simulink model "simulink_group17"  (R2023b)
settings: Solver=FixedStepAuto  StartTime=0.0  StopTime=10.0  FixedStep=1e-3  RelTol=1e-3  EnableMultiTasking=on
undefined symbols (not defined in the file): D0, D1, D10, D11, D12, D13, D2, D3, D4, D5, D6, D7, D8, D9, PTA0, PTA1, PTA2, PTB23, PTB9, PTC16, PTC17, PTC2, PTC3, PTC4, PTD0, PTD1, PTD2, PTD3
libraries: frdmk64flib x15
settings Model: ExtModeTrigDuration=5  Creator=ow  LastModifiedBy=reemb
settings SolverCC: AlgebraicLoopSolver=TrustRegion
settings OptimizationCC: EnhancedBackFolding=on  PassReuseOutputArgsAs=Individual arguments  ZeroExternalMemoryAtStartup=off  ZeroInternalMemoryAtStartup=off  MaxStackSize=64  OptimizeBlockOrder=speed  DifferentSizesBufferReuse=on  OptimizationCustomize=off  EfficientTunableParamExpr=on
settings DebuggingCC: ParameterTunabilityLossMsg=error  UnconnectedInputMsg=warning  UnconnectedOutputMsg=warning  UnconnectedLineMsg=warning
settings HardwareCC: ProdBitPerPointer=32  ProdBitPerSizeT=32  ProdBitPerPtrDiffT=32  ProdLargestAtomicInteger=Long  ProdLargestAtomicFloat=Double  ProdWordSize=32  ProdHWDeviceType=ARM Compatible->ARM Cortex
settings ModelReferenceCC: EnableRefExpFcnMdlSchedulingChecks=on
settings SFSimCC: MATLABDynamicMemAlloc=off
settings RTWCC: Description=Embedded Coder  SystemTargetFile=ert.tlc  HardwareBoard=NXP FRDM-K64F  TLCOptions="-aInlineSetEventsForThisBaseRateFcn=TLC_FALSE -aSuppressMultiTaskScheduler=TLC_FALSE  -aRateBasedStepFcn=0"  TemplateMakefile=ert_default_tmf  Toolchain=GNU Tools for ARM Embedded Processors
settings CodeAppCC: ForceParamTrailComments=on  IgnoreCustomStorageClasses=off  OperatorAnnotations=on  SimulinkDataObjDesc=on  SFDataObjDesc=on  InsertBlockDesc=on

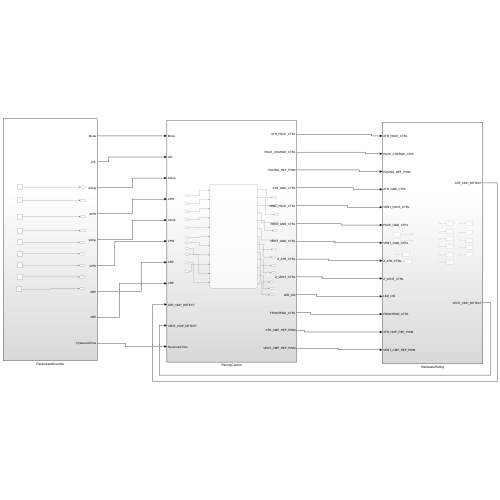
[thumbnail: Simulink's stored preview of the top-level diagram]
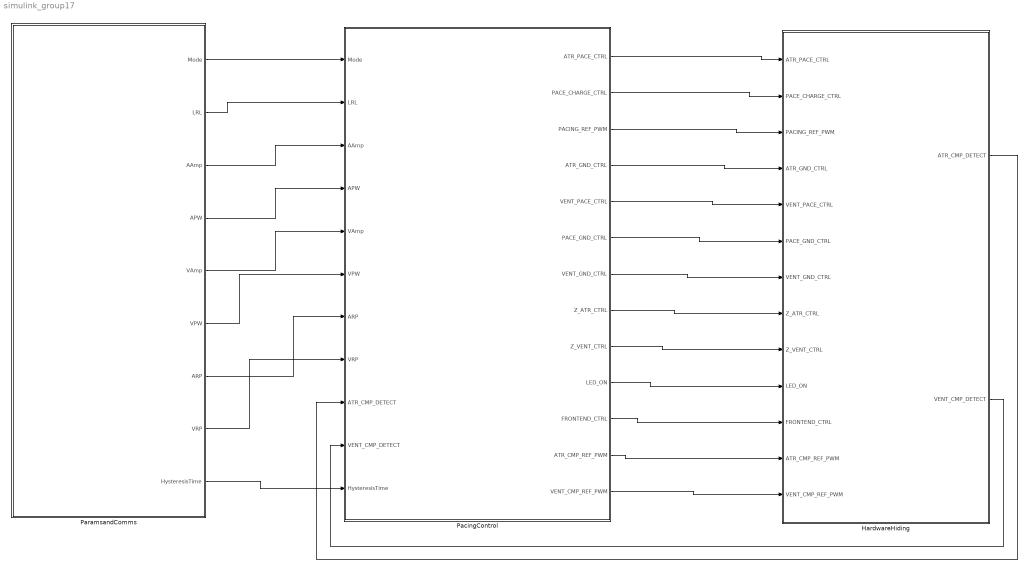
== system simulink_group17 ==
  HardwareHiding : Subsystem
  PacingControl : Subsystem
  ParamsandComms : Subsystem
  wires:
  ParamsandComms/1(Mode) -> PacingControl/1(Mode)
  ParamsandComms/2(LRL) -> PacingControl/2(LRL)
  ParamsandComms/3(AAmp) -> PacingControl/3(AAmp)
  ParamsandComms/4(APW) -> PacingControl/4(APW)
  ParamsandComms/6(VPW) -> PacingControl/6(VPW)
  ParamsandComms/5(VAmp) -> PacingControl/5(VAmp)
  ParamsandComms/7(ARP) -> PacingControl/7(ARP)
  ParamsandComms/8(VRP) -> PacingControl/8(VRP)
  PacingControl/1(ATR_PACE_CTRL) -> HardwareHiding/1(ATR_PACE_CTRL)
  PacingControl/2(PACE_CHARGE_CTRL) -> HardwareHiding/2(PACE_CHARGE_CTRL)
  PacingControl/3(PACING_REF_PWM) -> HardwareHiding/3(PACING_REF_PWM)
  PacingControl/5(VENT_PACE_CTRL) -> HardwareHiding/5(VENT_PACE_CTRL)
  PacingControl/4(ATR_GND_CTRL) -> HardwareHiding/4(ATR_GND_CTRL)
  PacingControl/6(PACE_GND_CTRL) -> HardwareHiding/6(PACE_GND_CTRL)
  PacingControl/7(VENT_GND_CTRL) -> HardwareHiding/7(VENT_GND_CTRL)
  PacingControl/8(Z_ATR_CTRL) -> HardwareHiding/8(Z_ATR_CTRL)
  PacingControl/9(Z_VENT_CTRL) -> HardwareHiding/9(Z_VENT_CTRL)
  PacingControl/10(LED_ON) -> HardwareHiding/10(LED_ON)
  PacingControl/11(FRONTEND_CTRL) -> HardwareHiding/11(FRONTEND_CTRL)
  ParamsandComms/9(HysteresisTime) -> PacingControl/11(HysteresisTime)
  HardwareHiding/1(ATR_CMP_DETECT) -> PacingControl/9(ATR_CMP_DETECT)
  HardwareHiding/2(VENT_CMP_DETECT) -> PacingControl/10(VENT_CMP_DETECT)
  PacingControl/12(ATR_CMP_REF_PWM) -> HardwareHiding/12(ATR_CMP_REF_PWM)
  PacingControl/13(VENT_CMP_REF_PWM) -> HardwareHiding/13(VENT_CMP_REF_PWM)

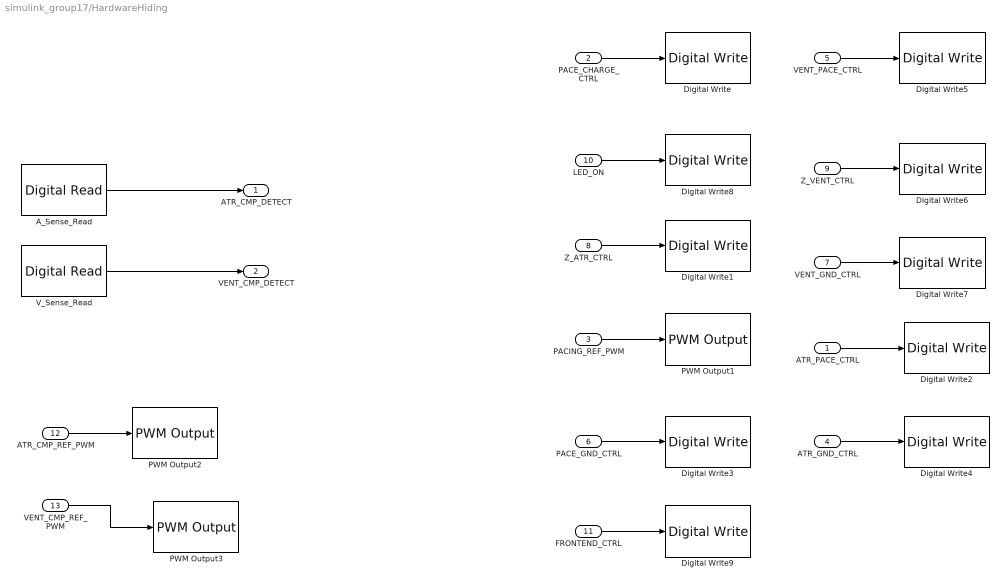
== system simulink_group17/HardwareHiding ==
  ATR_PACE_CTRL : Inport
  PACE_CHARGE_CTRL : Inport  Port=2
  PACING_REF_PWM : Inport  Port=3
  ATR_GND_CTRL : Inport  Port=4
  VENT_PACE_CTRL : Inport  Port=5
  PACE_GND_CTRL : Inport  Port=6
  VENT_GND_CTRL : Inport  Port=7
  Z_ATR_CTRL : Inport  Port=8
  Z_VENT_CTRL : Inport  Port=9
  LED_ON : Inport  Port=10
  FRONTEND_CTRL : Inport  Port=11
  ATR_CMP_REF_PWM : Inport  Port=12
  VENT_CMP_REF_PWM : Inport  Port=13
  A_Sense_Read : frdmk64flib/Digital Read  Whichpin=PTC16 (D0)  SampleTime=-1
  Digital Write : frdmk64flib/Digital Write  Whichpin=PTB9 (D2)
  Digital Write1 : frdmk64flib/Digital Write  Whichpin=PTB23 (D4)
  Digital Write2 : frdmk64flib/Digital Write  Whichpin=PTA0 (D8)
  Digital Write3 : frdmk64flib/Digital Write  Whichpin=PTD0 (D10)
  Digital Write4 : frdmk64flib/Digital Write  Whichpin=PTD2 (D11)
  Digital Write5 : frdmk64flib/Digital Write  Whichpin=PTC4 (D9)
  Digital Write6 : frdmk64flib/Digital Write  Whichpin=PTC3 (D7)
  Digital Write7 : frdmk64flib/Digital Write  Whichpin=PTD3 (D12)
  Digital Write8 : frdmk64flib/Digital Write  Whichpin=RED_LED
  Digital Write9 : frdmk64flib/Digital Write  Whichpin=PTD1 (D13)
  PWM Output1 : frdmk64flib/PWM Output  Whichpin=PTA2 (D5)  InitialFrequency=2000  InitialDutyCycle=50
  PWM Output2 : frdmk64flib/PWM Output  Whichpin=PTC2 (D6)  InitialFrequency=2000  InitialDutyCycle=100
  PWM Output3 : frdmk64flib/PWM Output  Whichpin=PTA1 (D3)  InitialFrequency=2000  InitialDutyCycle=100
  V_Sense_Read : frdmk64flib/Digital Read  Whichpin=PTC17 (D1)  SampleTime=-1
  ATR_CMP_DETECT : Outport
  VENT_CMP_DETECT : Outport  Port=2
  wires:
  A_Sense_Read/1 -> ATR_CMP_DETECT/1
  V_Sense_Read/1 -> VENT_CMP_DETECT/1
  Z_VENT_CTRL/1 -> Digital Write6/1
  LED_ON/1 -> Digital Write8/1
  ATR_PACE_CTRL/1 -> Digital Write2/1
  Z_ATR_CTRL/1 -> Digital Write1/1
  VENT_GND_CTRL/1 -> Digital Write7/1
  PACE_CHARGE_CTRL/1 -> Digital Write/1
  PACE_GND_CTRL/1 -> Digital Write3/1
  PACING_REF_PWM/1 -> PWM Output1/1
  VENT_PACE_CTRL/1 -> Digital Write5/1
  ATR_GND_CTRL/1 -> Digital Write4/1
  FRONTEND_CTRL/1 -> Digital Write9/1
  ATR_CMP_REF_PWM/1 -> PWM Output2/1
  VENT_CMP_REF_PWM/1 -> PWM Output3/1

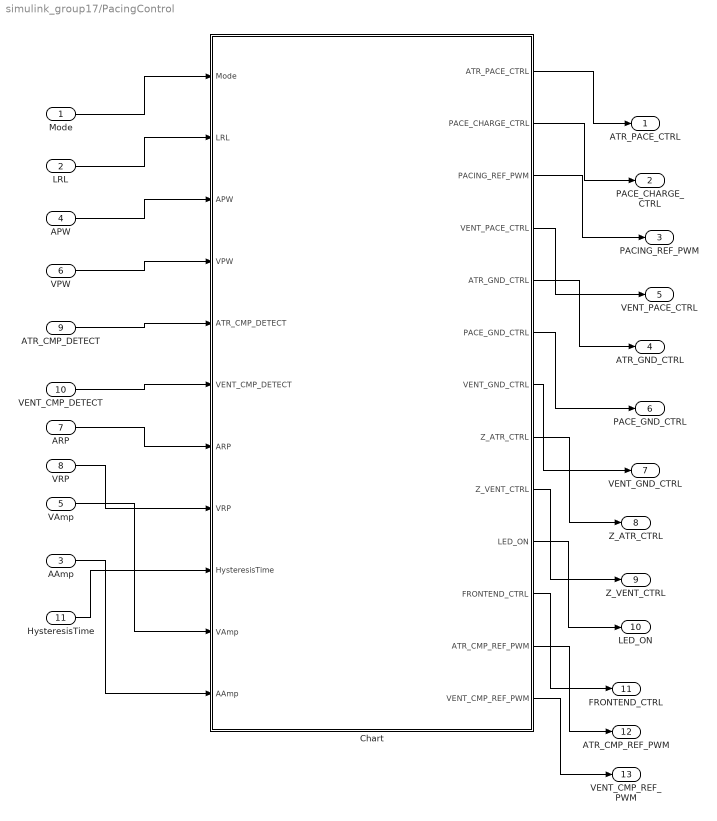
== system simulink_group17/PacingControl ==
  Mode : Inport
  LRL : Inport  Port=2
  AAmp : Inport  Port=3
  APW : Inport  Port=4
  VAmp : Inport  Port=5
  VPW : Inport  Port=6
  ARP : Inport  Port=7
  VRP : Inport  Port=8
  ATR_CMP_DETECT : Inport  Port=9
  VENT_CMP_DETECT : Inport  Port=10
  HysteresisTime : Inport  Port=11
  Chart : Stateflow chart  TreatAsAtomicUnit=on
      settings: PortSchema="{\"entries\":[{\"content\":{\"sides\":[{\"content\":{\"connectorIds\":[\"In1\",\"In2\",\"In5\",\"In3\",\"In4\",\"In6\",\"In7\",\"In10\",\"In11\",\"In8\",\"In9\"]},\"type\":\"ConnectorPlacement.EquallySpacedRectSide\",\"uuid\":\"2cabd690-10ca-439e-b217-62815d125176\"},{\"content\":{\"connectorIds\":[\"Out1\",\"Out2\",\"Out3\",\"Out4\",\"Out5\",\"Out6\",\"Out7\",\"Out8\",\"Out9\",\"Out10\",\"Out11\",\"Out12\",\"Out13\"],\"side\":\"RIGHT\"},\"type\":\"ConnectorPlacement.EquallySpacedRectSide\",\"uuid\":\"e8964e9d-7b02-47f5-a48a-30c87640778e\"},{\"content\":{\"side\":\"TOP\"},\"type\":\"ConnectorPlacement.EquallySpacedRectSide\",\"uuid\":\"37da63f5-52a1-4b9c-b728-2e179414b5fa\"}]},\"type\":\"ConnectorPlacement.EquallySpacedConnector\",\"uuid\":\"fe4480b5-e88f-4b9f-8d05-cd2d47a8a31d\"}],\"packageUris\":[\"http://schema.mathworks.com/mf0/Connector/R2020b\"],\"version\":\"1.0\"}"
  ATR_PACE_CTRL : Outport
  PACE_CHARGE_CTRL : Outport  Port=2
  PACING_REF_PWM : Outport  Port=3
  ATR_GND_CTRL : Outport  Port=4
  VENT_PACE_CTRL : Outport  Port=5
  PACE_GND_CTRL : Outport  Port=6
  VENT_GND_CTRL : Outport  Port=7
  Z_ATR_CTRL : Outport  Port=8
  Z_VENT_CTRL : Outport  Port=9
  LED_ON : Outport  Port=10
  FRONTEND_CTRL : Outport  Port=11
  ATR_CMP_REF_PWM : Outport  Port=12
  VENT_CMP_REF_PWM : Outport  Port=13
  wires:
  LRL/1 -> Chart/2(LRL)
  Mode/1 -> Chart/1(Mode)
  VPW/1 -> Chart/3(VPW)
  ATR_CMP_DETECT/1 -> Chart/4(ATR_CMP_DETECT)
  APW/1 -> Chart/5(APW)
  ARP/1 -> Chart/7(ARP)
  VRP/1 -> Chart/10(VRP)
  AAmp/1 -> Chart/9(AAmp)
  VAmp/1 -> Chart/8(VAmp)
  Chart/1(ATR_PACE_CTRL) -> ATR_PACE_CTRL/1
  Chart/2(PACE_CHARGE_CTRL) -> PACE_CHARGE_CTRL/1
  Chart/3(PACING_REF_PWM) -> PACING_REF_PWM/1
  Chart/5(ATR_GND_CTRL) -> ATR_GND_CTRL/1
  Chart/6(PACE_GND_CTRL) -> PACE_GND_CTRL/1
  Chart/7(VENT_GND_CTRL) -> VENT_GND_CTRL/1
  Chart/8(Z_ATR_CTRL) -> Z_ATR_CTRL/1
  Chart/9(Z_VENT_CTRL) -> Z_VENT_CTRL/1
  Chart/11(FRONTEND_CTRL) -> FRONTEND_CTRL/1
  HysteresisTime/1 -> Chart/11(HysteresisTime)
  Chart/4(VENT_PACE_CTRL) -> VENT_PACE_CTRL/1
  Chart/10(LED_ON) -> LED_ON/1
  VENT_CMP_DETECT/1 -> Chart/6(VENT_CMP_DETECT)
  Chart/12(ATR_CMP_REF_PWM) -> ATR_CMP_REF_PWM/1
  Chart/13(VENT_CMP_REF_PWM) -> VENT_CMP_REF_PWM/1

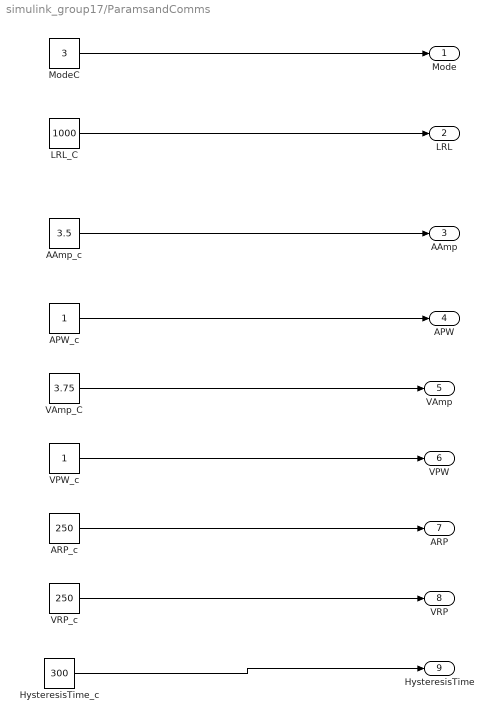
== system simulink_group17/ParamsandComms ==
  AAmp_c : Constant  Value=3.5
  APW_c : Constant
  ARP_c : Constant  Value=250
  HysteresisTime_c : Constant  Value=300
  LRL_C : Constant  Value=1000  SampleTime=-1
  ModeC : Constant  Value=3
  VAmp_C : Constant  Value=3.75
  VPW_c : Constant
  VRP_c : Constant  Value=250
  Mode : Outport
  LRL : Outport  Port=2
  AAmp : Outport  Port=3
  APW : Outport  Port=4
  VAmp : Outport  Port=5
  VPW : Outport  Port=6
  ARP : Outport  Port=7
  VRP : Outport  Port=8
  HysteresisTime : Outport  Port=9
  wires:
  ModeC/1 -> Mode/1
  LRL_C/1 -> LRL/1
  AAmp_c/1 -> AAmp/1
  APW_c/1 -> APW/1
  VRP_c/1 -> VRP/1
  ARP_c/1 -> ARP/1
  VPW_c/1 -> VPW/1
  VAmp_C/1 -> VAmp/1
  HysteresisTime_c/1 -> HysteresisTime/1

== stateflow chart simulink_group17/PacingControl/Chart ==
  state AAI
    state ChargingDischarging
      entry:
      %Enable Sensing
      FRONTEND_CTRL = 1;
      ATR_CMP_REF_PWM = 90;
      %Charging
      PACE_CHARGE_CTRL = 1;
      ATR_PACE_CTRL = 0;
      VENT_PACE_CTRL = 0;
      PACING_REF_PWM = (AAmp/5) * 100;
      %Discharging
      PACE_GND_CTRL = 1;
      ATR_PACE_CTRL = 0;
      ATR_GND_CTRL = 1;
      VENT_PACE_CTRL = 0;
      VENT_GND_CTRL = 0;
      Z_ATR_CTRL = 0;
      Z_VENT_CTRL = 0;
      LED_ON = 0;
    state Pacing
      entry:
      %Disable Sensing
      FRONTEND_CTRL = 0;
      %Pace Ventricle
      PACE_CHARGE_CTRL = 0;
      PACE_GND_CTRL = 1;
      ATR_PACE_CTRL = 1;
      ATR_GND_CTRL = 0;
      VENT_PACE_CTRL = 0;
      VENT_GND_CTRL = 0;
      Z_ATR_CTRL = 0;
      Z_VENT_CTRL = 0;
      LED_ON = 1;
    state Hysteresis
      entry:
      %Enable Sensing
      FRONTEND_CTRL = 1;
      %Charging
      PACE_CHARGE_CTRL = 1;
      ATR_PACE_CTRL = 0;
      VENT_PACE_CTRL = 0;
      %Discharging
      PACE_GND_CTRL = 1;
      ATR_PACE_CTRL = 0;
      ATR_GND_CTRL = 1;
      VENT_PACE_CTRL = 0;
      VENT_GND_CTRL = 0;
      Z_ATR_CTRL = 0;
      Z_VENT_CTRL = 0;
      LED_ON = 0;
    (default) -> AAI.ChargingDischarging
    AAI.ChargingDischarging -> AAI.Pacing [order 1] : [after(LRL- ARP, msec) ]
    AAI.Pacing -> AAI.ChargingDischarging : [after(APW,msec)]
    AAI.Hysteresis -> AAI.Pacing [order 2] : [after(LRL + HysteresisTime, msec)]
    AAI.Hysteresis -> AAI.ChargingDischarging [order 3] : [after(ARP, msec)]
    AAI.ChargingDischarging -> AAI.Hysteresis [order 2] : [ ATR_CMP_DETECT==1]
    AAI.Hysteresis -> AAI.Hysteresis [order 1] : [after(ARP, msec) && ATR_CMP_DETECT==1]
  state VVI
    state ChargingDischarging
      entry:
      %Enable Sensing
      FRONTEND_CTRL = 1;
      VENT_CMP_REF_PWM = 90;
      %Charging
      PACE_CHARGE_CTRL = 1;
      ATR_PACE_CTRL = 0;
      VENT_PACE_CTRL = 0;
      PACING_REF_PWM = (VAmp/5) * 100;
      %Discharging
      PACE_GND_CTRL = 1;
      ATR_PACE_CTRL = 0;
      ATR_GND_CTRL = 0;
      VENT_PACE_CTRL = 0;
      VENT_GND_CTRL = 1;
      Z_ATR_CTRL = 0;
      Z_VENT_CTRL = 0;
      LED_ON = 0;
    state VPacing
      entry:
      %Disable Sensing
      FRONTEND_CTRL = 0;
      %Pace Ventricle
      PACE_CHARGE_CTRL = 0;
      PACE_GND_CTRL = 1;
      ATR_PACE_CTRL = 0;
      ATR_GND_CTRL = 0;
      VENT_PACE_CTRL = 1;
      VENT_GND_CTRL = 0;
      Z_ATR_CTRL = 0;
      Z_VENT_CTRL = 0;
      LED_ON = 1;
    state Hysteresis
      entry:
      %Enable Sensing
      FRONTEND_CTRL = 1;
      %Charging
      PACE_CHARGE_CTRL = 1;
      ATR_PACE_CTRL = 0;
      VENT_PACE_CTRL = 0;
      %Discharging
      PACE_GND_CTRL = 1;
      ATR_PACE_CTRL = 0;
      ATR_GND_CTRL = 0;
      VENT_PACE_CTRL = 0;
      VENT_GND_CTRL = 1;
      Z_ATR_CTRL = 0;
      Z_VENT_CTRL = 0;
      LED_ON = 0;
    (default) -> VVI.ChargingDischarging
    VVI.ChargingDischarging -> VVI.VPacing [order 1] : [after(LRL-VRP, msec) ]
    VVI.VPacing -> VVI.ChargingDischarging : [after(VPW,msec)]
    VVI.Hysteresis -> VVI.VPacing [order 2] : [after(LRL + HysteresisTime, msec)]
    VVI.Hysteresis -> VVI.ChargingDischarging [order 3] : [after(VRP, msec)]
    VVI.ChargingDischarging -> VVI.Hysteresis [order 2] : [ VENT_CMP_DETECT==1]
    VVI.Hysteresis -> VVI.Hysteresis [order 1] : [after(VRP, msec) && VENT_CMP_DETECT==1]
  state AOO
    state APacing
      entry:
      %Pace Atrial
      PACE_CHARGE_CTRL = 0;
      PACE_GND_CTRL = 1;
      ATR_PACE_CTRL = 1;
      ATR_GND_CTRL = 0;
      VENT_PACE_CTRL = 0;
      VENT_GND_CTRL = 0;
      Z_ATR_CTRL = 0;
      Z_VENT_CTRL = 0;
      LED_ON = 1;
    state ChargingDischarging
      entry:
      %No Sensing
      FRONTEND_CTRL = 0;
      %Charging
      PACE_CHARGE_CTRL = 1;
      ATR_PACE_CTRL = 0;
      VENT_PACE_CTRL = 0;
      PACING_REF_PWM = (AAmp/5) * 100;
      %Discharging
      PACE_GND_CTRL = 1;
      ATR_PACE_CTRL = 0;
      ATR_GND_CTRL = 1;
      VENT_PACE_CTRL = 0;
      VENT_GND_CTRL = 0;
      Z_ATR_CTRL = 0;
      Z_VENT_CTRL = 0;
      LED_ON = 0;
    (default) -> state26
    AOO.APacing -> state26 : [after(APW,msec)]
    state26 -> AOO.APacing : [after(LRL-APW,msec)]
  state VOO
    state Chargin_Discharging
      entry:
      %No Sensing
      FRONTEND_CTRL = 0;
      %Charging
      PACE_CHARGE_CTRL = 1;
      ATR_PACE_CTRL = 0;
      VENT_PACE_CTRL = 0;
      PACING_REF_PWM = (VAmp/5) * 100;
      %Discharging
      PACE_GND_CTRL = 1;
      ATR_PACE_CTRL = 0;
      ATR_GND_CTRL = 0;
      VENT_PACE_CTRL = 0;
      VENT_GND_CTRL = 1;
      Z_ATR_CTRL = 0;
      Z_VENT_CTRL = 0;
      LED_ON = 0;
    state Pacing
      entry:
      %Pace Ventricle
      PACE_CHARGE_CTRL = 0;
      PACE_GND_CTRL = 1;
      ATR_PACE_CTRL = 0;
      ATR_GND_CTRL = 0;
      VENT_PACE_CTRL = 1;
      VENT_GND_CTRL = 0;
      Z_ATR_CTRL = 0;
      Z_VENT_CTRL = 0;
      LED_ON = 1;
    (default) -> VOO.Chargin_Discharging
    VOO.Chargin_Discharging -> VOO.Pacing : [after(LRL-VPW,msec)]
    VOO.Pacing -> VOO.Chargin_Discharging : [after(VPW,msec)]
  state InitialState
  state VVIR
    state ChargingDischarging
      entry:
      %Enable Sensing
      FRONTEND_CTRL = 1;
      VENT_CMP_REF_PWM = 90;
      %Charging
      PACE_CHARGE_CTRL = 1;
      ATR_PACE_CTRL = 0;
      VENT_PACE_CTRL = 0;
      PACING_REF_PWM = (VAmp/5) * 100;
      %Discharging
      PACE_GND_CTRL = 1;
      ATR_PACE_CTRL = 0;
      ATR_GND_CTRL = 0;
      VENT_PACE_CTRL = 0;
      VENT_GND_CTRL = 1;
      Z_ATR_CTRL = 0;
      Z_VENT_CTRL = 0;
      LED_ON = 0;
    state VPacing
      entry:
      %Disable Sensing
      FRONTEND_CTRL = 0;
      %Pace Ventricle
      PACE_CHARGE_CTRL = 0;
      PACE_GND_CTRL = 1;
      ATR_PACE_CTRL = 0;
      ATR_GND_CTRL = 0;
      VENT_PACE_CTRL = 1;
      VENT_GND_CTRL = 0;
      Z_ATR_CTRL = 0;
      Z_VENT_CTRL = 0;
      LED_ON = 1;
    state Hysteresis
      entry:
      %Enable Sensing
      FRONTEND_CTRL = 1;
      %Charging
      PACE_CHARGE_CTRL = 1;
      ATR_PACE_CTRL = 0;
      VENT_PACE_CTRL = 0;
      %Discharging
      PACE_GND_CTRL = 1;
      ATR_PACE_CTRL = 0;
      ATR_GND_CTRL = 0;
      VENT_PACE_CTRL = 0;
      VENT_GND_CTRL = 1;
      Z_ATR_CTRL = 0;
      Z_VENT_CTRL = 0;
      LED_ON = 0;
    (default) -> VVIR.ChargingDischarging
    VVIR.ChargingDischarging -> VVIR.VPacing [order 1] : [after(LRL-VRP, msec) ]
    VVIR.VPacing -> VVIR.ChargingDischarging : [after(VPW,msec)]
    VVIR.Hysteresis -> VVIR.VPacing [order 2] : [after(LRL + HysteresisTime, msec)]
    VVIR.Hysteresis -> VVIR.ChargingDischarging [order 3] : [after(VRP, msec)]
    VVIR.ChargingDischarging -> VVIR.Hysteresis [order 2] : [ VENT_CMP_DETECT==1]
    VVIR.Hysteresis -> VVIR.Hysteresis [order 1] : [after(VRP, msec) && VENT_CMP_DETECT==1]
  state AOOR
    state APacing
      entry:
      %Pace Atrial
      PACE_CHARGE_CTRL = 0;
      PACE_GND_CTRL = 1;
      ATR_PACE_CTRL = 1;
      ATR_GND_CTRL = 0;
      VENT_PACE_CTRL = 0;
      VENT_GND_CTRL = 0;
      Z_ATR_CTRL = 0;
      Z_VENT_CTRL = 0;
      LED_ON = 1;
    state ChargingDischarging
      entry:
      %No Sensing
      FRONTEND_CTRL = 0;
      %Charging
      PACE_CHARGE_CTRL = 1;
      ATR_PACE_CTRL = 0;
      VENT_PACE_CTRL = 0;
      PACING_REF_PWM = (AAmp/5) * 100;
      %Discharging
      PACE_GND_CTRL = 1;
      ATR_PACE_CTRL = 0;
      ATR_GND_CTRL = 1;
      VENT_PACE_CTRL = 0;
      VENT_GND_CTRL = 0;
      Z_ATR_CTRL = 0;
      Z_VENT_CTRL = 0;
      LED_ON = 0;
    note: % Switch out LRL in the transition with wtvr accelerometer variable you have (for all 4 new modes)
    (default) -> AOOR.ChargingDischarging
    AOOR.APacing -> AOOR.ChargingDischarging : [after(APW,msec)]
    AOOR.ChargingDischarging -> AOOR.APacing : [after(LRL-APW,msec)]
  state AAIR
    state ChargingDischarging
      entry:
      %Enable Sensing
      FRONTEND_CTRL = 1;
      ATR_CMP_REF_PWM = 90;
      %Charging
      PACE_CHARGE_CTRL = 1;
      ATR_PACE_CTRL = 0;
      VENT_PACE_CTRL = 0;
      PACING_REF_PWM = (AAmp/5) * 100;
      %Discharging
      PACE_GND_CTRL = 1;
      ATR_PACE_CTRL = 0;
      ATR_GND_CTRL = 1;
      VENT_PACE_CTRL = 0;
      VENT_GND_CTRL = 0;
      Z_ATR_CTRL = 0;
      Z_VENT_CTRL = 0;
      LED_ON = 0;
    state Pacing
      entry:
      %Disable Sensing
      FRONTEND_CTRL = 0;
      %Pace Ventricle
      PACE_CHARGE_CTRL = 0;
      PACE_GND_CTRL = 1;
      ATR_PACE_CTRL = 1;
      ATR_GND_CTRL = 0;
      VENT_PACE_CTRL = 0;
      VENT_GND_CTRL = 0;
      Z_ATR_CTRL = 0;
      Z_VENT_CTRL = 0;
      LED_ON = 1;
    state Hysteresis
      entry:
      %Enable Sensing
      FRONTEND_CTRL = 1;
      %Charging
      PACE_CHARGE_CTRL = 1;
      ATR_PACE_CTRL = 0;
      VENT_PACE_CTRL = 0;
      %Discharging
      PACE_GND_CTRL = 1;
      ATR_PACE_CTRL = 0;
      ATR_GND_CTRL = 1;
      VENT_PACE_CTRL = 0;
      VENT_GND_CTRL = 0;
      Z_ATR_CTRL = 0;
      Z_VENT_CTRL = 0;
      LED_ON = 0;
    (default) -> AAIR.ChargingDischarging
    AAIR.ChargingDischarging -> AAIR.Pacing [order 1] : [after(LRL- ARP, msec) ]
    AAIR.Pacing -> AAIR.ChargingDischarging : [after(APW,msec)]
    AAIR.Hysteresis -> AAIR.Pacing [order 2] : [after(LRL + HysteresisTime, msec)]
    AAIR.Hysteresis -> AAIR.ChargingDischarging [order 3] : [after(ARP, msec)]
    AAIR.ChargingDischarging -> AAIR.Hysteresis [order 2] : [ ATR_CMP_DETECT==1]
    AAIR.Hysteresis -> AAIR.Hysteresis [order 1] : [after(ARP, msec) && ATR_CMP_DETECT==1]
  state VOOR
    state Chargin_Discharging
      entry:
      %No Sensing
      FRONTEND_CTRL = 0;
      %Charging
      PACE_CHARGE_CTRL = 1;
      ATR_PACE_CTRL = 0;
      VENT_PACE_CTRL = 0;
      PACING_REF_PWM = (VAmp/5) * 100;
      %Discharging
      PACE_GND_CTRL = 1;
      ATR_PACE_CTRL = 0;
      ATR_GND_CTRL = 0;
      VENT_PACE_CTRL = 0;
      VENT_GND_CTRL = 1;
      Z_ATR_CTRL = 0;
      Z_VENT_CTRL = 0;
      LED_ON = 0;
    state Pacing
      entry:
      %Pace Ventricle
      PACE_CHARGE_CTRL = 0;
      PACE_GND_CTRL = 1;
      ATR_PACE_CTRL = 0;
      ATR_GND_CTRL = 0;
      VENT_PACE_CTRL = 1;
      VENT_GND_CTRL = 0;
      Z_ATR_CTRL = 0;
      Z_VENT_CTRL = 0;
      LED_ON = 1;
    (default) -> VOOR.Chargin_Discharging
    VOOR.Chargin_Discharging -> VOOR.Pacing : [after(LRL-VPW,msec)]
    VOOR.Pacing -> VOOR.Chargin_Discharging : [after(VPW,msec)]
  InitialState -> VVI [order 4] : [Mode==4]
  InitialState -> AAI [order 3] : [Mode==3]
  InitialState -> VOO [order 2] : [Mode==2]
  InitialState -> AOO [order 1] : [Mode==1]
  (default) -> InitialState
  InitialState -> AOOR [order 5] : [Mode==5]
  InitialState -> VOOR [order 6] : [Mode==6]
  InitialState -> AAIR [order 7] : [Mode==7]
  InitialState -> VVIR [order 8] : [Mode==8]
  data: Mode input; LRL input; VPW input; ATR_CMP_DETECT input; APW input; VENT_CMP_DETECT input; ARP input; VAmp input; AAmp input; VRP input; ATR_PACE_CTRL output; PACE_CHARGE_CTRL output; PACING_REF_PWM output; VENT_PACE_CTRL output; ATR_GND_CTRL output; PACE_GND_CTRL output; VENT_GND_CTRL output; Z_ATR_CTRL output; Z_VENT_CTRL output; LED_ON output; FRONTEND_CTRL output; HysteresisTime input; ATR_CMP_REF_PWM output; VENT_CMP_REF_PWM output
